simulink subsystem "s3x3_ULA_additive_Noise_Interference"  (R2020b)
settings: Solver=VariableStepAuto  StartTime=0.0  StopTime=10.0  RelTol=1e-3
values from neighbouring files (symbols this model uses):
  fc = 30e6    (= 30000000)    [env_sim_setup.m]
  finf = 200e6    (= 200000000)    [env_sim_setup.m]
  fs = 1e9    (= 1000000000)    [env_sim_setup.m]
  noiseP = 1    [env_sim_setup.m]
  phShftD = (0:1:N-1)*eAngD    [env_sim_setup.m]
  phShftI = (0:1:N-1)*eAngI    [env_sim_setup.m]
  SNR = 1    [env_sim_setup.m]
  sv = sv - 0.0001*1i    [env_sim_setup.m]
undefined symbols (not defined in the file or in its folder): datetime, second
libraries: dspsrcs4 x6, simulink x1
settings Model: Creator=jgentile  LastModifiedBy=jgentile

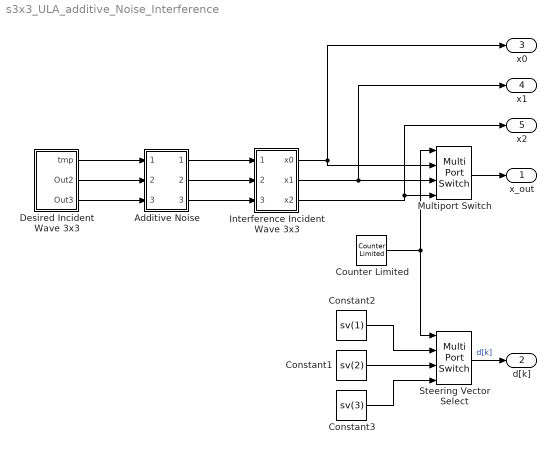
== system s3x3_ULA_additive_Noise_Interference ==
  Additive Noise : Subsystem
  Constant1 : Constant  Value=sv(2)
  Constant2 : Constant  Value=sv(1)
  Constant3 : Constant  Value=sv(3)
  Counter Limited : simulink/Sources/Counter Limited  uplimit=2  tsamp=-1
  Desired Incident Wave 3x3 : Subsystem
  Interference Incident Wave 3x3 : Subsystem
  Multiport Switch : MultiPortSwitch  DataPortOrder=Zero-based contiguous  zeroidx=on
  Steering Vector Select : MultiPortSwitch  DataPortOrder=Zero-based contiguous  zeroidx=on
  x_out : Outport
  d[k] : Outport  Port=2
      settings: SignalType=complex
  x0 : Outport  Port=3
  x1 : Outport  Port=4
  x2 : Outport  Port=5
  wires:
  Constant1/1 -> Steering Vector Select/3
  Constant3/1 -> Steering Vector Select/4
  Multiport Switch/1 -> x_out/1
  Steering Vector Select/1 -> d[k]/1  "d[k]"
  Counter Limited/1 -> Multiport Switch/1, Steering Vector Select/1
  Constant2/1 -> Steering Vector Select/2
  Desired Incident Wave 3x3/1(tmp) -> Additive Noise/1(In1)
  Desired Incident Wave 3x3/2(Out2) -> Additive Noise/2(In2)
  Desired Incident Wave 3x3/3(Out3) -> Additive Noise/3(In3)
  Additive Noise/1(Input) -> Interference Incident Wave 3x3/1(Input)
  Additive Noise/2(Input1) -> Interference Incident Wave 3x3/2(Input1)
  Additive Noise/3(Input2) -> Interference Incident Wave 3x3/3(Input2)
  Interference Incident Wave 3x3/3(x2) -> Multiport Switch/4, x2/1
  Interference Incident Wave 3x3/2(x1) -> Multiport Switch/3, x1/1
  Interference Incident Wave 3x3/1(x0) -> Multiport Switch/2, x0/1

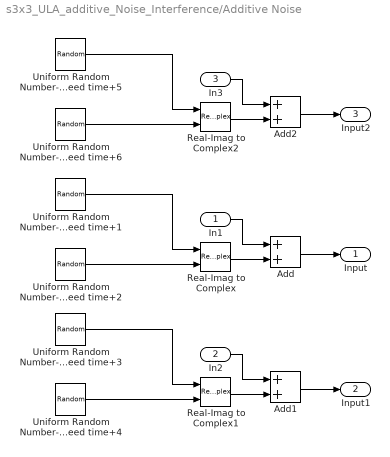
== system s3x3_ULA_additive_Noise_Interference/Additive Noise ==
  In1 : Inport
  In2 : Inport  Port=2
  In3 : Inport  Port=3
  Add : Sum
  Add1 : Sum
  Add2 : Sum
  Real-Imag to Complex : RealImagToComplex
  Real-Imag to Complex1 : RealImagToComplex
  Real-Imag to Complex2 : RealImagToComplex
  Uniform Random Number- Seed time+1 : UniformRandomNumber  Minimum=-sqrt(SNR*noiseP)  Maximum=sqrt(SNR*noiseP)  Seed=round(second(datetime('now')))+1  SampleTime=1/fs
  Uniform Random Number- Seed time+2 : UniformRandomNumber  Minimum=-sqrt(SNR*noiseP)  Maximum=sqrt(SNR*noiseP)  Seed=round(second(datetime('now')))+2  SampleTime=1/fs
  Uniform Random Number- Seed time+3 : UniformRandomNumber  Minimum=-sqrt(SNR*noiseP)  Maximum=sqrt(SNR*noiseP)  Seed=round(second(datetime('now')))+3  SampleTime=1/fs
  Uniform Random Number- Seed time+4 : UniformRandomNumber  Minimum=-sqrt(SNR*noiseP)  Maximum=sqrt(SNR*noiseP)  Seed=round(second(datetime('now')))+4  SampleTime=1/fs
  Uniform Random Number- Seed time+5 : UniformRandomNumber  Minimum=-sqrt(SNR*noiseP)  Maximum=sqrt(SNR*noiseP)  Seed=round(second(datetime('now')))+5  SampleTime=1/fs
  Uniform Random Number- Seed time+6 : UniformRandomNumber  Minimum=-sqrt(SNR*noiseP)  Maximum=sqrt(SNR*noiseP)  Seed=round(second(datetime('now')))+6  SampleTime=1/fs
  Input : Outport
  Input1 : Outport  Port=2
  Input2 : Outport  Port=3
  wires:
  Add/1 -> Input/1
  Uniform Random Number- Seed time+5/1 -> Real-Imag to Complex2/1
  Real-Imag to Complex2/1 -> Add2/2
  Add2/1 -> Input2/1
  Uniform Random Number- Seed time+4/1 -> Real-Imag to Complex1/2
  In3/1 -> Add2/1
  Real-Imag to Complex/1 -> Add/2
  Uniform Random Number- Seed time+3/1 -> Real-Imag to Complex1/1
  In1/1 -> Add/1
  Add1/1 -> Input1/1
  Uniform Random Number- Seed time+2/1 -> Real-Imag to Complex/2
  In2/1 -> Add1/1
  Uniform Random Number- Seed time+1/1 -> Real-Imag to Complex/1
  Uniform Random Number- Seed time+6/1 -> Real-Imag to Complex2/2
  Real-Imag to Complex1/1 -> Add1/2

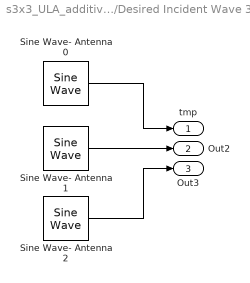
== system s3x3_ULA_additive_Noise_Interference/Desired Incident Wave 3x3 ==
  Sine Wave- Antenna 0 : dspsrcs4/Sine Wave  Amplitude=SNR  Frequency=fc  Phase=phShftD(1)  SampleMode=Discrete  OutComplex=Complex  CompMethod=Trigonometric fcn  TableSize=Speed  SampleTime=1/fs  SamplesPerFrame=1  ResetState=Restart at time zero  OutputFrames=off  dataType=double  wordLen=16  udDataType=sfix(16)  fracBitsMode=Best precision  numFracBits=15  OutDataTypeStr=double  LastOutDataTypeStr=double
  Sine Wave- Antenna 1 : dspsrcs4/Sine Wave  Amplitude=SNR  Frequency=fc  Phase=phShftD(2)  SampleMode=Discrete  OutComplex=Complex  CompMethod=Trigonometric fcn  TableSize=Speed  SampleTime=1/fs  SamplesPerFrame=1  ResetState=Restart at time zero  OutputFrames=off  dataType=double  wordLen=16  udDataType=sfix(16)  fracBitsMode=Best precision  numFracBits=15  OutDataTypeStr=double  LastOutDataTypeStr=double
  Sine Wave- Antenna 2 : dspsrcs4/Sine Wave  Amplitude=SNR  Frequency=fc  Phase=phShftD(3)  SampleMode=Discrete  OutComplex=Complex  CompMethod=Trigonometric fcn  TableSize=Speed  SampleTime=1/fs  SamplesPerFrame=1  ResetState=Restart at time zero  OutputFrames=off  dataType=double  wordLen=16  udDataType=sfix(16)  fracBitsMode=Best precision  numFracBits=15  OutDataTypeStr=double  LastOutDataTypeStr=double
  tmp : Outport
  Out2 : Outport  Port=2
  Out3 : Outport  Port=3
  wires:
  Sine Wave- Antenna 1/1 -> Out2/1
  Sine Wave- Antenna 0/1 -> tmp/1
  Sine Wave- Antenna 2/1 -> Out3/1

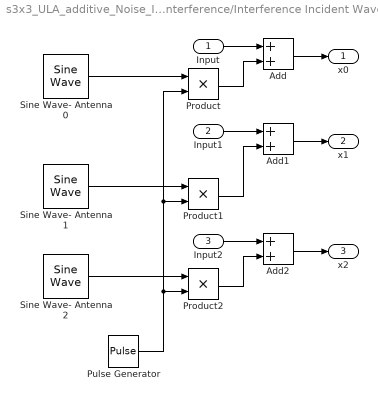
== system s3x3_ULA_additive_Noise_Interference/Interference Incident Wave 3x3 ==
  Input : Inport
  Input1 : Inport  Port=2
  Input2 : Inport  Port=3
  Add : Sum
  Add1 : Sum
  Add2 : Sum
  Product : Product
  Product1 : Product
  Product2 : Product
  Pulse Generator : DiscretePulseGenerator  Period=10000  PulseWidth=2000  PhaseDelay=3000  SampleTime=1/fs
  Sine Wave- Antenna 0 : dspsrcs4/Sine Wave  Amplitude=4*SNR  Frequency=finf  Phase=phShftI(1)  SampleMode=Discrete  OutComplex=Complex  CompMethod=Trigonometric fcn  TableSize=Speed  SampleTime=1/fs  SamplesPerFrame=1  ResetState=Restart at time zero  OutputFrames=off  dataType=double  wordLen=16  udDataType=sfix(16)  fracBitsMode=Best precision  numFracBits=15  OutDataTypeStr=double  LastOutDataTypeStr=double
  Sine Wave- Antenna 1 : dspsrcs4/Sine Wave  Amplitude=4*SNR  Frequency=finf  Phase=phShftI(2)  SampleMode=Discrete  OutComplex=Complex  CompMethod=Trigonometric fcn  TableSize=Speed  SampleTime=1/fs  SamplesPerFrame=1  ResetState=Restart at time zero  OutputFrames=off  dataType=double  wordLen=16  udDataType=sfix(16)  fracBitsMode=Best precision  numFracBits=15  OutDataTypeStr=double  LastOutDataTypeStr=double
  Sine Wave- Antenna 2 : dspsrcs4/Sine Wave  Amplitude=4*SNR  Frequency=finf  Phase=phShftI(3)  SampleMode=Discrete  OutComplex=Complex  CompMethod=Trigonometric fcn  TableSize=Speed  SampleTime=1/fs  SamplesPerFrame=1  ResetState=Restart at time zero  OutputFrames=off  dataType=double  wordLen=16  udDataType=sfix(16)  fracBitsMode=Best precision  numFracBits=15  OutDataTypeStr=double  LastOutDataTypeStr=double
  x0 : Outport
  x1 : Outport  Port=2
  x2 : Outport  Port=3
  wires:
  Pulse Generator/1 -> Product2/2, Product1/2, Product/2
  Product2/1 -> Add2/2
  Product1/1 -> Add1/2
  Product/1 -> Add/2
  Sine Wave- Antenna 1/1 -> Product1/1
  Sine Wave- Antenna 0/1 -> Product/1
  Input2/1 -> Add2/1
  Sine Wave- Antenna 2/1 -> Product2/1
  Input1/1 -> Add1/1
  Add1/1 -> x1/1
  Add/1 -> x0/1
  Add2/1 -> x2/1
  Input/1 -> Add/1
